simulink model "TflexDriver"  (R2018a)
settings: Solver=FixedStepAuto  StartTime=0.0  StopTime=inf  FixedStep=ts  RelTol=1e-3  EnableMultiTasking=on
values from neighbouring files (symbols this model uses):
  ts = 1/1000    (= 0.001)    [Tflex_PID_init.m]    (also in init.m = 0.00025; multisineInit.m)
libraries: xpcethercatlib x91, simulink x60
(part 1 of 2)
settings Model: SimulationMode=external  Creator=wout7  LastModifiedBy=wout7
settings SolverCC: ConcurrentTasks=on  AutoInsertRateTranBlk=on
settings DataIOCC: SaveFormat=StructureWithTime
settings OptimizationCC: BlockReduction=off  OptimizeBlockIOStorage=off  BufferReuse=off  GlobalBufferReuse=off  ExpressionFolding=off  LocalBlockOutputs=off  OptimizeDataStoreBuffers=off  BusAssignmentInplaceUpdate=off
settings HardwareCC: ProdBitPerPointer=32  ProdBitPerSizeT=32  ProdBitPerPtrDiffT=32  ProdLargestAtomicFloat=None  ProdWordSize=32  ProdLongLongMode=on  ProdHWDeviceType=Generic->32-bit x86 compatible
settings RTWCC: SystemTargetFile=slrt.tlc  TemplateMakefile=slrt_default_tmf  Description=Simulink Real-Time  CodeExecutionProfiling=on  RTWCompilerOptimization=on
settings SimulinkRealTimeCC: SupportVariableSizeSignals=on  RL32LogTETModifier=off  xPCConcurrentTasks=on

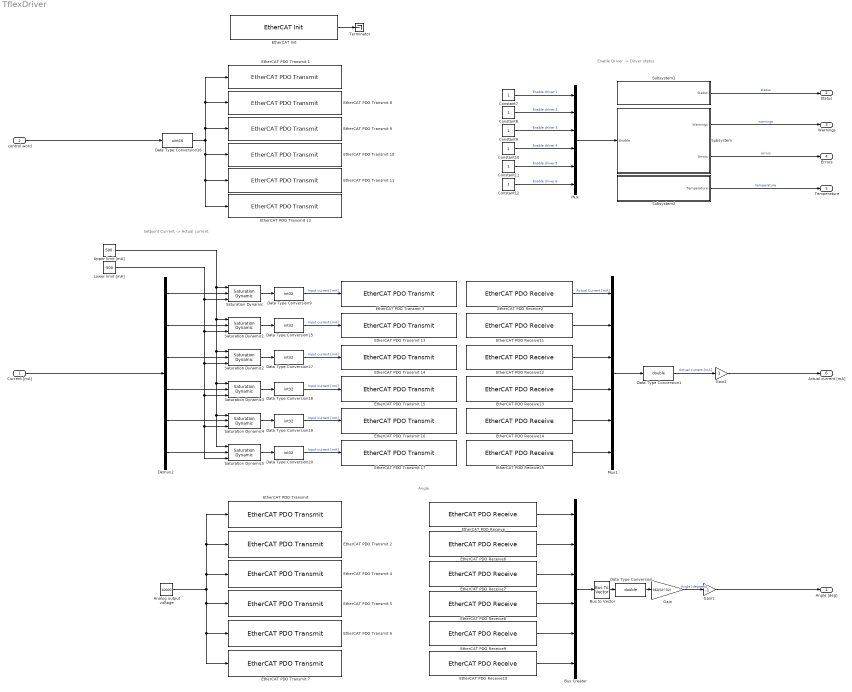
== system TflexDriver ==
  note: Angle
  note: Setpoint Current -> Actual current
  note: Enable Driver -> Dirver status
  Current [mA] : Inport
  control word : Inport  Port=2
  Analog output voltage : Constant  Value=10000  OutDataTypeStr=int16  SampleTime=-1
  Bus Creator : BusCreator  Inputs=6
  Bus to Vector : BusToVector
  Constant{7..12} (6 alike) : Constant  OutDataTypeStr=int32  SampleTime=1
  Data Type Conversion : DataTypeConversion  OutDataTypeStr=double
  Data Type Conversion1 : DataTypeConversion  OutDataTypeStr=double
  Data Type Conversion{9,15,17..20} (6 alike) : DataTypeConversion  OutDataTypeStr=int32
  Data Type Conversion16 : DataTypeConversion  OutDataTypeStr=uint16
  Demux2 : Demux  Outputs=6
  "EtherCAT Init " : xpcethercatlib/EtherCAT Init   Priority=0  config_file=C:\Users\wout7\Documents\GitHub\Inverse_dynamics_learning\TargetPC\6 DOF\pdo_mapping_6dr_1kHz.xml  device_id=0  pci_bus=13  pci_slot=0  pci_function=0  dctuning=0  enaDebug=off  enaDC=on  errLink=off  masterDbg=off  stateChgDbg=off  baseClock=off  masterCfg=off  logFile='c:\dbglog.txt'  sample_time=0.001000  DCMode=2
      settings: SourceProductName=Simulink Real-Time  SourceProductBaseCode=XP
  EtherCAT PDO Receive : xpcethercatlib/EtherCAT PDO Receive  Priority=2  sig_name=Drive 2 (AKD).Inputs_1.Position actual internal value  sig_offset=560  sig_type=int32  type_size=32  sig_dim=1  device_id=0  sample_time=0.001000
      settings: SourceProductName=Simulink Real-Time  SourceProductBaseCode=XP
  EtherCAT PDO Receive10 : xpcethercatlib/EtherCAT PDO Receive  Priority=2  sig_name=Drive 7 (AKD).Inputs_1.Position actual internal value  sig_offset=37488  sig_type=int32  type_size=32  sig_dim=1  device_id=0  sample_time=0.001000
      settings: SourceProductName=Simulink Real-Time  SourceProductBaseCode=XP
  EtherCAT PDO Receive11 : xpcethercatlib/EtherCAT PDO Receive  Priority=2  sig_name=Drive 3 (AKD).Inputs_1.Current actual value  sig_offset=12560  sig_type=int32  type_size=32  sig_dim=1  device_id=0  sample_time=0.001000
      settings: SourceProductName=Simulink Real-Time  SourceProductBaseCode=XP
  EtherCAT PDO Receive12 : xpcethercatlib/EtherCAT PDO Receive  Priority=2  sig_name=Drive 4 (AKD).Inputs_1.Current actual value  sig_offset=24848  sig_type=int32  type_size=32  sig_dim=1  device_id=0  sample_time=0.001000
      settings: SourceProductName=Simulink Real-Time  SourceProductBaseCode=XP
  EtherCAT PDO Receive13 : xpcethercatlib/EtherCAT PDO Receive  Priority=2  sig_name=Drive 5 (AKD).Inputs_1.Current actual value  sig_offset=37136  sig_type=int32  type_size=32  sig_dim=1  device_id=0  sample_time=0.001000
      settings: SourceProductName=Simulink Real-Time  SourceProductBaseCode=XP
  EtherCAT PDO Receive14 : xpcethercatlib/EtherCAT PDO Receive  Priority=2  sig_name=Drive 6 (AKD).Inputs_1.Current actual value  sig_offset=37296  sig_type=int32  type_size=32  sig_dim=1  device_id=0  sample_time=0.001000
      settings: SourceProductName=Simulink Real-Time  SourceProductBaseCode=XP
  EtherCAT PDO Receive15 : xpcethercatlib/EtherCAT PDO Receive  Priority=2  sig_name=Drive 7 (AKD).Inputs_1.Current actual value  sig_offset=37456  sig_type=int32  type_size=32  sig_dim=1  device_id=0  sample_time=0.001000
      settings: SourceProductName=Simulink Real-Time  SourceProductBaseCode=XP
  EtherCAT PDO Receive2 : xpcethercatlib/EtherCAT PDO Receive  Priority=2  sig_name=Drive 2 (AKD).Inputs_1.Current actual value  sig_offset=528  sig_type=int32  type_size=32  sig_dim=1  device_id=0  sample_time=0.001000
      settings: SourceProductName=Simulink Real-Time  SourceProductBaseCode=XP
  EtherCAT PDO Receive6 : xpcethercatlib/EtherCAT PDO Receive  Priority=2  sig_name=Drive 3 (AKD).Inputs_1.Position actual internal value  sig_offset=12592  sig_type=int32  type_size=32  sig_dim=1  device_id=0  sample_time=0.001000
      settings: SourceProductName=Simulink Real-Time  SourceProductBaseCode=XP
  EtherCAT PDO Receive7 : xpcethercatlib/EtherCAT PDO Receive  Priority=2  sig_name=Drive 4 (AKD).Inputs_1.Position actual internal value  sig_offset=24880  sig_type=int32  type_size=32  sig_dim=1  device_id=0  sample_time=0.001000
      settings: SourceProductName=Simulink Real-Time  SourceProductBaseCode=XP
  EtherCAT PDO Receive8 : xpcethercatlib/EtherCAT PDO Receive  Priority=2  sig_name=Drive 5 (AKD).Inputs_1.Position actual internal value  sig_offset=37168  sig_type=int32  type_size=32  sig_dim=1  device_id=0  sample_time=0.001000
      settings: SourceProductName=Simulink Real-Time  SourceProductBaseCode=XP
  EtherCAT PDO Receive9 : xpcethercatlib/EtherCAT PDO Receive  Priority=2  sig_name=Drive 6 (AKD).Inputs_1.Position actual internal value  sig_offset=37328  sig_type=int32  type_size=32  sig_dim=1  device_id=0  sample_time=0.001000
      settings: SourceProductName=Simulink Real-Time  SourceProductBaseCode=XP
  "EtherCAT PDO Transmit " : xpcethercatlib/EtherCAT PDO Transmit   Priority=3  sig_name=Drive 2 (AKD).Outputs.AOUT.VALUE write  sig_offset=480  sig_type=int16  type_size=16  sig_dim=1  device_id=0  sample_time=0.001000
      settings: SourceProductName=Simulink Real-Time  SourceProductBaseCode=XP
  EtherCAT PDO Transmit 1 : xpcethercatlib/EtherCAT PDO Transmit   Priority=3  sig_name=Drive 2 (AKD).Outputs.Controlword  sig_offset=464  sig_type=uint16  type_size=16  sig_dim=1  device_id=0  sample_time=0.001000
      settings: SourceProductName=Simulink Real-Time  SourceProductBaseCode=XP
  EtherCAT PDO Transmit 10 : xpcethercatlib/EtherCAT PDO Transmit   Priority=3  sig_name=Drive 5 (AKD).Outputs.Controlword  sig_offset=37072  sig_type=uint16  type_size=16  sig_dim=1  device_id=0  sample_time=0.001000
      settings: SourceProductName=Simulink Real-Time  SourceProductBaseCode=XP
  EtherCAT PDO Transmit 11 : xpcethercatlib/EtherCAT PDO Transmit   Priority=3  sig_name=Drive 6 (AKD).Outputs.Controlword  sig_offset=37232  sig_type=uint16  type_size=16  sig_dim=1  device_id=0  sample_time=0.001000
      settings: SourceProductName=Simulink Real-Time  SourceProductBaseCode=XP
  EtherCAT PDO Transmit 12 : xpcethercatlib/EtherCAT PDO Transmit   Priority=3  sig_name=Drive 7 (AKD).Outputs.Controlword  sig_offset=37392  sig_type=uint16  type_size=16  sig_dim=1  device_id=0  sample_time=0.001000
      settings: SourceProductName=Simulink Real-Time  SourceProductBaseCode=XP
  EtherCAT PDO Transmit 13 : xpcethercatlib/EtherCAT PDO Transmit   Priority=3  sig_name=Drive 3 (AKD).Outputs.Target current  sig_offset=12528  sig_type=int32  type_size=32  sig_dim=1  device_id=0  sample_time=0.001000
      settings: SourceProductName=Simulink Real-Time  SourceProductBaseCode=XP
  EtherCAT PDO Transmit 14 : xpcethercatlib/EtherCAT PDO Transmit   Priority=3  sig_name=Drive 4 (AKD).Outputs.Target current  sig_offset=24816  sig_type=int32  type_size=32  sig_dim=1  device_id=0  sample_time=0.001000
      settings: SourceProductName=Simulink Real-Time  SourceProductBaseCode=XP
  EtherCAT PDO Transmit 15 : xpcethercatlib/EtherCAT PDO Transmit   Priority=3  sig_name=Drive 5 (AKD).Outputs.Target current  sig_offset=37104  sig_type=int32  type_size=32  sig_dim=1  device_id=0  sample_time=0.001000
      settings: SourceProductName=Simulink Real-Time  SourceProductBaseCode=XP
  EtherCAT PDO Transmit 16 : xpcethercatlib/EtherCAT PDO Transmit   Priority=3  sig_name=Drive 6 (AKD).Outputs.Target current  sig_offset=37264  sig_type=int32  type_size=32  sig_dim=1  device_id=0  sample_time=0.001000
      settings: SourceProductName=Simulink Real-Time  SourceProductBaseCode=XP
  EtherCAT PDO Transmit 17 : xpcethercatlib/EtherCAT PDO Transmit   Priority=3  sig_name=Drive 7 (AKD).Outputs.Target current  sig_offset=37424  sig_type=int32  type_size=32  sig_dim=1  device_id=0  sample_time=0.001000
      settings: SourceProductName=Simulink Real-Time  SourceProductBaseCode=XP
  EtherCAT PDO Transmit 2 : xpcethercatlib/EtherCAT PDO Transmit   Priority=3  sig_name=Drive 3 (AKD).Outputs.AOUT.VALUE write  sig_offset=12512  sig_type=int16  type_size=16  sig_dim=1  device_id=0  sample_time=0.001000
      settings: SourceProductName=Simulink Real-Time  SourceProductBaseCode=XP
  EtherCAT PDO Transmit 3 : xpcethercatlib/EtherCAT PDO Transmit   Priority=3  sig_name=Drive 2 (AKD).Outputs.Target current  sig_offset=496  sig_type=int32  type_size=32  sig_dim=1  device_id=0  sample_time=0.001000
      settings: SourceProductName=Simulink Real-Time  SourceProductBaseCode=XP
  EtherCAT PDO Transmit 4 : xpcethercatlib/EtherCAT PDO Transmit   Priority=3  sig_name=Drive 4 (AKD).Outputs.AOUT.VALUE write  sig_offset=24800  sig_type=int16  type_size=16  sig_dim=1  device_id=0  sample_time=0.001000
      settings: SourceProductName=Simulink Real-Time  SourceProductBaseCode=XP
  EtherCAT PDO Transmit 5 : xpcethercatlib/EtherCAT PDO Transmit   Priority=3  sig_name=Drive 5 (AKD).Outputs.AOUT.VALUE write  sig_offset=37088  sig_type=int16  type_size=16  sig_dim=1  device_id=0  sample_time=0.001000
      settings: SourceProductName=Simulink Real-Time  SourceProductBaseCode=XP
  EtherCAT PDO Transmit 6 : xpcethercatlib/EtherCAT PDO Transmit   Priority=3  sig_name=Drive 6 (AKD).Outputs.AOUT.VALUE write  sig_offset=37248  sig_type=int16  type_size=16  sig_dim=1  device_id=0  sample_time=0.001000
      settings: SourceProductName=Simulink Real-Time  SourceProductBaseCode=XP
  EtherCAT PDO Transmit 7 : xpcethercatlib/EtherCAT PDO Transmit   Priority=3  sig_name=Drive 7 (AKD).Outputs.AOUT.VALUE write  sig_offset=37408  sig_type=int16  type_size=16  sig_dim=1  device_id=0  sample_time=0.001000
      settings: SourceProductName=Simulink Real-Time  SourceProductBaseCode=XP
  EtherCAT PDO Transmit 8 : xpcethercatlib/EtherCAT PDO Transmit   Priority=3  sig_name=Drive 3 (AKD).Outputs.Controlword  sig_offset=12496  sig_type=uint16  type_size=16  sig_dim=1  device_id=0  sample_time=0.001000
      settings: SourceProductName=Simulink Real-Time  SourceProductBaseCode=XP
  EtherCAT PDO Transmit 9 : xpcethercatlib/EtherCAT PDO Transmit   Priority=3  sig_name=Drive 4 (AKD).Outputs.Controlword  sig_offset=24784  sig_type=uint16  type_size=16  sig_dim=1  device_id=0  sample_time=0.001000
      settings: SourceProductName=Simulink Real-Time  SourceProductBaseCode=XP
  Gain : Gain  Gain=360/(2^32)
  Gain1 : Gain  Gain=-1
  Gain2 : Gain
  Lower limit [mA] : Constant  Value=-500  SampleTime=ts
  Mux : Mux  Inputs=6
  Mux1 : Mux  Inputs=6
  Saturation Dynamic{,1..5} (6 alike) : simulink/Discontinuities/Saturation Dynamic  OutMin=[]  OutMax=[]  OutDataTypeStr=Inherit: Same as second input  OutDataType=fixdt(1, 16)  OutScaling=2^-10  DoSatur=off
  Subsystem : Subsystem
  Subsystem1 : Subsystem
  Subsystem2 : Subsystem
  Terminator : Terminator
  Upper limit [mA] : Constant  Value=500  SampleTime=ts
  Angle [deg] : Outport
  Status : Outport  Port=2
  Warnings : Outport  Port=3
  Errors : Outport  Port=4
  Temperature : Outport  Port=5
  Actual current [mA] : Outport  Port=6
  wires:
  Lower limit [mA]/1 -> Saturation Dynamic/3, Saturation Dynamic1/3, Saturation Dynamic2/3, Saturation Dynamic3/3, Saturation Dynamic4/3, Saturation Dynamic5/3
  Data Type Conversion17/1 -> EtherCAT PDO Transmit 14/1  "Input current [mA]"
  Data Type Conversion/1 -> Gain/1
  Constant7/1 -> Mux/1  "Enable driver 1"
  EtherCAT PDO Receive10/1 -> Bus Creator/6
  Analog output voltage/1 -> EtherCAT PDO Transmit 7/1, EtherCAT PDO Transmit 6/1, EtherCAT PDO Transmit 5/1, "EtherCAT PDO Transmit "/1, EtherCAT PDO Transmit 2/1, EtherCAT PDO Transmit 4/1
  Subsystem1/1(Status) -> Status/1  "status"
  Constant12/1 -> Mux/6  "Enable driver 6"
  EtherCAT PDO Receive2/1 -> Mux1/1  "Actual Current [mA]"
  Mux/1 -> Subsystem/1(Enable)
  Subsystem/1(Warnings) -> Warnings/1  "warnings"
  Saturation Dynamic1/1 -> Data Type Conversion15/1
  EtherCAT PDO Receive11/1 -> Mux1/2
  Gain1/1 -> Angle [deg]/1
  Gain2/1 -> Actual current [mA]/1
  control word/1 -> Data Type Conversion16/1
  Current [mA]/1 -> Demux2/1
  Data Type Conversion16/1 -> EtherCAT PDO Transmit 1/1, EtherCAT PDO Transmit 8/1, EtherCAT PDO Transmit 9/1, EtherCAT PDO Transmit 12/1, EtherCAT PDO Transmit 11/1, EtherCAT PDO Transmit 10/1
  Gain/1 -> Gain1/1  "Angle [degrees]"
  Subsystem2/1(Temperature) -> Temperature/1  "temperature"
  Demux2/6 -> Saturation Dynamic5/2
  Demux2/3 -> Saturation Dynamic2/2
  Saturation Dynamic5/1 -> Data Type Conversion20/1
  Demux2/2 -> Saturation Dynamic1/2
  Upper limit [mA]/1 -> Saturation Dynamic3/1, Saturation Dynamic4/1, Saturation Dynamic5/1, Saturation Dynamic2/1, Saturation Dynamic1/1, Saturation Dynamic/1
  Saturation Dynamic2/1 -> Data Type Conversion17/1
  Bus to Vector/1 -> Data Type Conversion/1
  Mux1/1 -> Data Type Conversion1/1
  Constant9/1 -> Mux/3  "Enable driver 3"
  Data Type Conversion15/1 -> EtherCAT PDO Transmit 13/1  "Input current [mA]"
  Data Type Conversion19/1 -> EtherCAT PDO Transmit 16/1  "Input current [mA]"
  EtherCAT PDO Receive7/1 -> Bus Creator/3
  Data Type Conversion20/1 -> EtherCAT PDO Transmit 17/1  "Input current [mA]"
  EtherCAT PDO Receive/1 -> Bus Creator/1
  Demux2/5 -> Saturation Dynamic4/2
  Bus Creator/1 -> Bus to Vector/1
  Data Type Conversion1/1 -> Gain2/1  "Actual current [mA]"
  EtherCAT PDO Receive14/1 -> Mux1/5
  Constant10/1 -> Mux/4  "Enable driver 4"
  Constant11/1 -> Mux/5  "Enable driver 5"
  Demux2/1 -> Saturation Dynamic/2
  EtherCAT PDO Receive9/1 -> Bus Creator/5
  Data Type Conversion9/1 -> EtherCAT PDO Transmit 3/1  "Input current [mA]"
  Constant8/1 -> Mux/2  "Enable driver 2"
  EtherCAT PDO Receive13/1 -> Mux1/4
  EtherCAT PDO Receive12/1 -> Mux1/3
  Saturation Dynamic4/1 -> Data Type Conversion19/1
  Demux2/4 -> Saturation Dynamic3/2
  Data Type Conversion18/1 -> EtherCAT PDO Transmit 15/1  "Input current [mA]"
  EtherCAT PDO Receive6/1 -> Bus Creator/2
  EtherCAT PDO Receive8/1 -> Bus Creator/4
  EtherCAT PDO Receive15/1 -> Mux1/6
  Subsystem/2(Errors) -> Errors/1  "errors"
  Saturation Dynamic/1 -> Data Type Conversion9/1
  "EtherCAT Init "/1 -> Terminator/1
  Saturation Dynamic3/1 -> Data Type Conversion18/1

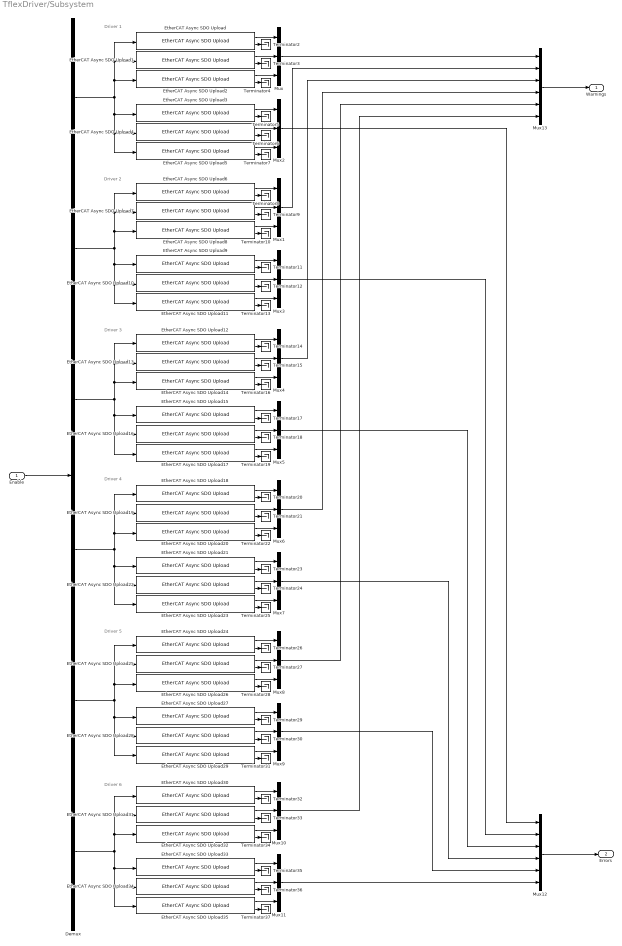
== system TflexDriver/Subsystem ==
  note: Driver 1
  note: Driver 2
  note: Driver 3
  note: Driver 4
  note: Driver 5
  note: Driver 6
  Enable : Inport
  Demux : Demux  Outputs=6
  EtherCAT Async SDO Upload : xpcethercatlib/EtherCAT Async SDO Upload  index=8192  subIndex=1  sig_type=uint32  sig_dim=1  device_id=0  slave_name=Drive 2 (AKD)  sample_time=1  slave_addr=1001  selected_slave=Term 1 (EK1100)  timeout=500  slave_found=1
      settings: SourceProductName=Simulink Real-Time  SourceProductBaseCode=XP
  EtherCAT Async SDO Upload1 : xpcethercatlib/EtherCAT Async SDO Upload  index=8192  subIndex=2  sig_type=uint32  sig_dim=1  device_id=0  slave_name=Drive 2 (AKD)  sample_time=1  slave_addr=1001  selected_slave=Term 1 (EK1100)  timeout=500  slave_found=1
      settings: SourceProductName=Simulink Real-Time  SourceProductBaseCode=XP
  EtherCAT Async SDO Upload10 : xpcethercatlib/EtherCAT Async SDO Upload  index=8193  subIndex=2  sig_type=uint32  sig_dim=1  device_id=0  slave_name=Drive 3 (AKD)  sample_time=1  slave_addr=1002  selected_slave=Term 1 (EK1100)  timeout=500  slave_found=1
      settings: SourceProductName=Simulink Real-Time  SourceProductBaseCode=XP
  EtherCAT Async SDO Upload11 : xpcethercatlib/EtherCAT Async SDO Upload  index=8193  subIndex=3  sig_type=uint32  sig_dim=1  device_id=0  slave_name=Drive 3 (AKD)  sample_time=1  slave_addr=1002  selected_slave=Term 1 (EK1100)  timeout=500  slave_found=1
      settings: SourceProductName=Simulink Real-Time  SourceProductBaseCode=XP
  EtherCAT Async SDO Upload12 : xpcethercatlib/EtherCAT Async SDO Upload  index=8192  subIndex=1  sig_type=uint32  sig_dim=1  device_id=0  slave_name=Drive 4 (AKD)  sample_time=1  slave_addr=1003  selected_slave=Term 1 (EK1100)  timeout=500  slave_found=1
      settings: SourceProductName=Simulink Real-Time  SourceProductBaseCode=XP
  EtherCAT Async SDO Upload13 : xpcethercatlib/EtherCAT Async SDO Upload  index=8192  subIndex=2  sig_type=uint32  sig_dim=1  device_id=0  slave_name=Drive 4 (AKD)  sample_time=1  slave_addr=1003  selected_slave=Term 1 (EK1100)  timeout=500  slave_found=1
      settings: SourceProductName=Simulink Real-Time  SourceProductBaseCode=XP
  EtherCAT Async SDO Upload14 : xpcethercatlib/EtherCAT Async SDO Upload  index=8192  subIndex=3  sig_type=uint32  sig_dim=1  device_id=0  slave_name=Drive 4 (AKD)  sample_time=1  slave_addr=1003  selected_slave=Term 1 (EK1100)  timeout=500  slave_found=1
      settings: SourceProductName=Simulink Real-Time  SourceProductBaseCode=XP
  EtherCAT Async SDO Upload15 : xpcethercatlib/EtherCAT Async SDO Upload  index=8193  subIndex=1  sig_type=uint32  sig_dim=1  device_id=0  slave_name=Drive 4 (AKD)  sample_time=1  slave_addr=1003  selected_slave=Term 1 (EK1100)  timeout=500  slave_found=1
      settings: SourceProductName=Simulink Real-Time  SourceProductBaseCode=XP
  EtherCAT Async SDO Upload16 : xpcethercatlib/EtherCAT Async SDO Upload  index=8193  subIndex=2  sig_type=uint32  sig_dim=1  device_id=0  slave_name=Drive 4 (AKD)  sample_time=1  slave_addr=1003  selected_slave=Term 1 (EK1100)  timeout=500  slave_found=1
      settings: SourceProductName=Simulink Real-Time  SourceProductBaseCode=XP
  EtherCAT Async SDO Upload17 : xpcethercatlib/EtherCAT Async SDO Upload  index=8193  subIndex=3  sig_type=uint32  sig_dim=1  device_id=0  slave_name=Drive 4 (AKD)  sample_time=1  slave_addr=1003  selected_slave=Term 1 (EK1100)  timeout=500  slave_found=1
      settings: SourceProductName=Simulink Real-Time  SourceProductBaseCode=XP
  EtherCAT Async SDO Upload18 : xpcethercatlib/EtherCAT Async SDO Upload  index=8192  subIndex=1  sig_type=uint32  sig_dim=1  device_id=0  slave_name=Drive 5 (AKD)  sample_time=1  slave_addr=1004  selected_slave=Term 1 (EK1100)  timeout=500  slave_found=1
      settings: SourceProductName=Simulink Real-Time  SourceProductBaseCode=XP
  EtherCAT Async SDO Upload19 : xpcethercatlib/EtherCAT Async SDO Upload  index=8192  subIndex=2  sig_type=uint32  sig_dim=1  device_id=0  slave_name=Drive 5 (AKD)  sample_time=1  slave_addr=1004  selected_slave=Term 1 (EK1100)  timeout=500  slave_found=1
      settings: SourceProductName=Simulink Real-Time  SourceProductBaseCode=XP
  EtherCAT Async SDO Upload2 : xpcethercatlib/EtherCAT Async SDO Upload  index=8192  subIndex=3  sig_type=uint32  sig_dim=1  device_id=0  slave_name=Drive 1 (AKD)  sample_time=1  slave_addr=1001  selected_slave=Term 1 (EK1100)  timeout=500  slave_found=1
      settings: SourceProductName=Simulink Real-Time  SourceProductBaseCode=XP
  EtherCAT Async SDO Upload20 : xpcethercatlib/EtherCAT Async SDO Upload  index=8192  subIndex=3  sig_type=uint32  sig_dim=1  device_id=0  slave_name=Drive 5 (AKD)  sample_time=1  slave_addr=1004  selected_slave=Term 1 (EK1100)  timeout=500  slave_found=1
      settings: SourceProductName=Simulink Real-Time  SourceProductBaseCode=XP
  EtherCAT Async SDO Upload21 : xpcethercatlib/EtherCAT Async SDO Upload  index=8193  subIndex=1  sig_type=uint32  sig_dim=1  device_id=0  slave_name=Drive 5 (AKD)  sample_time=1  slave_addr=1004  selected_slave=Term 1 (EK1100)  timeout=500  slave_found=1
      settings: SourceProductName=Simulink Real-Time  SourceProductBaseCode=XP
  EtherCAT Async SDO Upload22 : xpcethercatlib/EtherCAT Async SDO Upload  index=8193  subIndex=2  sig_type=uint32  sig_dim=1  device_id=0  slave_name=Drive 5 (AKD)  sample_time=1  slave_addr=1004  selected_slave=Term 1 (EK1100)  timeout=500  slave_found=1
      settings: SourceProductName=Simulink Real-Time  SourceProductBaseCode=XP
  EtherCAT Async SDO Upload23 : xpcethercatlib/EtherCAT Async SDO Upload  index=8193  subIndex=3  sig_type=uint32  sig_dim=1  device_id=0  slave_name=Drive 5 (AKD)  sample_time=1  slave_addr=1004  selected_slave=Term 1 (EK1100)  timeout=500  slave_found=1
      settings: SourceProductName=Simulink Real-Time  SourceProductBaseCode=XP
  EtherCAT Async SDO Upload24 : xpcethercatlib/EtherCAT Async SDO Upload  index=8192  subIndex=1  sig_type=uint32  sig_dim=1  device_id=0  slave_name=Drive 6 (AKD)  sample_time=1  slave_addr=1005  selected_slave=Term 1 (EK1100)  timeout=500  slave_found=1
      settings: SourceProductName=Simulink Real-Time  SourceProductBaseCode=XP
  EtherCAT Async SDO Upload25 : xpcethercatlib/EtherCAT Async SDO Upload  index=8192  subIndex=2  sig_type=uint32  sig_dim=1  device_id=0  slave_name=Drive 6 (AKD)  sample_time=1  slave_addr=1005  selected_slave=Term 1 (EK1100)  timeout=500  slave_found=1
      settings: SourceProductName=Simulink Real-Time  SourceProductBaseCode=XP
  EtherCAT Async SDO Upload26 : xpcethercatlib/EtherCAT Async SDO Upload  index=8192  subIndex=3  sig_type=uint32  sig_dim=1  device_id=0  slave_name=Drive 6 (AKD)  sample_time=1  slave_addr=1005  selected_slave=Term 1 (EK1100)  timeout=500  slave_found=1
      settings: SourceProductName=Simulink Real-Time  SourceProductBaseCode=XP
  EtherCAT Async SDO Upload27 : xpcethercatlib/EtherCAT Async SDO Upload  index=8193  subIndex=1  sig_type=uint32  sig_dim=1  device_id=0  slave_name=Drive 6 (AKD)  sample_time=1  slave_addr=1005  selected_slave=Term 1 (EK1100)  timeout=500  slave_found=1
      settings: SourceProductName=Simulink Real-Time  SourceProductBaseCode=XP
  EtherCAT Async SDO Upload28 : xpcethercatlib/EtherCAT Async SDO Upload  index=8193  subIndex=2  sig_type=uint32  sig_dim=1  device_id=0  slave_name=Drive 6 (AKD)  sample_time=1  slave_addr=1005  selected_slave=Term 1 (EK1100)  timeout=500  slave_found=1
      settings: SourceProductName=Simulink Real-Time  SourceProductBaseCode=XP
  EtherCAT Async SDO Upload29 : xpcethercatlib/EtherCAT Async SDO Upload  index=8193  subIndex=3  sig_type=uint32  sig_dim=1  device_id=0  slave_name=Drive 6 (AKD)  sample_time=1  slave_addr=1005  selected_slave=Term 1 (EK1100)  timeout=500  slave_found=1
      settings: SourceProductName=Simulink Real-Time  SourceProductBaseCode=XP
  EtherCAT Async SDO Upload3 : xpcethercatlib/EtherCAT Async SDO Upload  index=8193  subIndex=1  sig_type=uint32  sig_dim=1  device_id=0  slave_name=""  sample_time=1  slave_addr=0  selected_slave=Term 1 (EK1100)  timeout=500  slave_found=1
      settings: SourceProductName=Simulink Real-Time  SourceProductBaseCode=XP
  EtherCAT Async SDO Upload30 : xpcethercatlib/EtherCAT Async SDO Upload  index=8192  subIndex=1  sig_type=uint32  sig_dim=1  device_id=0  slave_name=Drive 7 (AKD)  sample_time=1  slave_addr=1006  selected_slave=Term 1 (EK1100)  timeout=500  slave_found=1
      settings: SourceProductName=Simulink Real-Time  SourceProductBaseCode=XP
  EtherCAT Async SDO Upload31 : xpcethercatlib/EtherCAT Async SDO Upload  index=8192  subIndex=2  sig_type=uint32  sig_dim=1  device_id=0  slave_name=Drive 7 (AKD)  sample_time=1  slave_addr=1006  selected_slave=Term 1 (EK1100)  timeout=500  slave_found=1
      settings: SourceProductName=Simulink Real-Time  SourceProductBaseCode=XP
  EtherCAT Async SDO Upload32 : xpcethercatlib/EtherCAT Async SDO Upload  index=8192  subIndex=3  sig_type=uint32  sig_dim=1  device_id=0  slave_name=Drive 7 (AKD)  sample_time=1  slave_addr=1006  selected_slave=Term 1 (EK1100)  timeout=500  slave_found=1
      settings: SourceProductName=Simulink Real-Time  SourceProductBaseCode=XP
  EtherCAT Async SDO Upload33 : xpcethercatlib/EtherCAT Async SDO Upload  index=8193  subIndex=1  sig_type=uint32  sig_dim=1  device_id=0  slave_name=Drive 7 (AKD)  sample_time=1  slave_addr=1006  selected_slave=Term 1 (EK1100)  timeout=500  slave_found=1
      settings: SourceProductName=Simulink Real-Time  SourceProductBaseCode=XP
  EtherCAT Async SDO Upload34 : xpcethercatlib/EtherCAT Async SDO Upload  index=8193  subIndex=2  sig_type=uint32  sig_dim=1  device_id=0  slave_name=Drive 7 (AKD)  sample_time=1  slave_addr=1006  selected_slave=Term 1 (EK1100)  timeout=500  slave_found=1
      settings: SourceProductName=Simulink Real-Time  SourceProductBaseCode=XP
  EtherCAT Async SDO Upload35 : xpcethercatlib/EtherCAT Async SDO Upload  index=8193  subIndex=3  sig_type=uint32  sig_dim=1  device_id=0  slave_name=Drive 7 (AKD)  sample_time=1  slave_addr=1006  selected_slave=Term 1 (EK1100)  timeout=500  slave_found=1
      settings: SourceProductName=Simulink Real-Time  SourceProductBaseCode=XP
  EtherCAT Async SDO Upload4 : xpcethercatlib/EtherCAT Async SDO Upload  index=8193  subIndex=2  sig_type=uint32  sig_dim=1  device_id=0  slave_name=Drive 2 (AKD)  sample_time=1  slave_addr=1001  selected_slave=Term 1 (EK1100)  timeout=500  slave_found=1
      settings: SourceProductName=Simulink Real-Time  SourceProductBaseCode=XP
  EtherCAT Async SDO Upload5 : xpcethercatlib/EtherCAT Async SDO Upload  index=8193  subIndex=3  sig_type=uint32  sig_dim=1  device_id=0  slave_name=Drive 1 (AKD)  sample_time=1  slave_addr=1001  selected_slave=Term 1 (EK1100)  timeout=500  slave_found=1
      settings: SourceProductName=Simulink Real-Time  SourceProductBaseCode=XP
  EtherCAT Async SDO Upload6 : xpcethercatlib/EtherCAT Async SDO Upload  index=8192  subIndex=1  sig_type=uint32  sig_dim=1  device_id=0  slave_name=Drive 3 (AKD)  sample_time=1  slave_addr=1002  selected_slave=Term 1 (EK1100)  timeout=500  slave_found=1
      settings: SourceProductName=Simulink Real-Time  SourceProductBaseCode=XP
  EtherCAT Async SDO Upload7 : xpcethercatlib/EtherCAT Async SDO Upload  index=8192  subIndex=2  sig_type=uint32  sig_dim=1  device_id=0  slave_name=Drive 3 (AKD)  sample_time=1  slave_addr=1002  selected_slave=Term 1 (EK1100)  timeout=500  slave_found=1
      settings: SourceProductName=Simulink Real-Time  SourceProductBaseCode=XP
  EtherCAT Async SDO Upload8 : xpcethercatlib/EtherCAT Async SDO Upload  index=8192  subIndex=3  sig_type=uint32  sig_dim=1  device_id=0  slave_name=Drive 3 (AKD)  sample_time=1  slave_addr=1002  selected_slave=Term 1 (EK1100)  timeout=500  slave_found=1
      settings: SourceProductName=Simulink Real-Time  SourceProductBaseCode=XP
  EtherCAT Async SDO Upload9 : xpcethercatlib/EtherCAT Async SDO Upload  index=8193  subIndex=1  sig_type=uint32  sig_dim=1  device_id=0  slave_name=Drive 3 (AKD)  sample_time=1  slave_addr=1002  selected_slave=Term 1 (EK1100)  timeout=500  slave_found=1
      settings: SourceProductName=Simulink Real-Time  SourceProductBaseCode=XP
  Mux{,1..11} (12 alike) : Mux  Inputs=3
  Mux12 : Mux  Inputs=6
  Mux13 : Mux  Inputs=6
  Terminator{2..37} (36 alike) : Terminator
  Warnings : Outport
  Errors : Outport  Port=2
  wires:
  EtherCAT Async SDO Upload13/2 -> Terminator15/1
  EtherCAT Async SDO Upload23/2 -> Terminator25/1
  EtherCAT Async SDO Upload25/2 -> Terminator27/1
  EtherCAT Async SDO Upload9/2 -> Terminator11/1
  EtherCAT Async SDO Upload5/2 -> Terminator7/1
  EtherCAT Async SDO Upload30/2 -> Terminator32/1
  EtherCAT Async SDO Upload27/2 -> Terminator29/1
  EtherCAT Async SDO Upload12/2 -> Terminator14/1
  EtherCAT Async SDO Upload24/2 -> Terminator26/1
  EtherCAT Async SDO Upload26/2 -> Terminator28/1
  Mux4/1 -> Mux13/3
  Demux/3 -> EtherCAT Async SDO Upload12/1, EtherCAT Async SDO Upload13/1, EtherCAT Async SDO Upload14/1, EtherCAT Async SDO Upload17/1, EtherCAT Async SDO Upload16/1, EtherCAT Async SDO Upload15/1
  EtherCAT Async SDO Upload30/1 -> Mux10/1
  Demux/2 -> EtherCAT Async SDO Upload11/1, EtherCAT Async SDO Upload10/1, EtherCAT Async SDO Upload9/1, EtherCAT Async SDO Upload6/1, EtherCAT Async SDO Upload7/1, EtherCAT Async SDO Upload8/1
  EtherCAT Async SDO Upload9/1 -> Mux3/1
  EtherCAT Async SDO Upload18/2 -> Terminator20/1
  EtherCAT Async SDO Upload8/2 -> Terminator10/1
  EtherCAT Async SDO Upload11/2 -> Terminator13/1
  Demux/6 -> EtherCAT Async SDO Upload30/1, EtherCAT Async SDO Upload31/1, EtherCAT Async SDO Upload32/1, EtherCAT Async SDO Upload35/1, EtherCAT Async SDO Upload34/1, EtherCAT Async SDO Upload33/1
  Demux/4 -> EtherCAT Async SDO Upload18/1, EtherCAT Async SDO Upload19/1, EtherCAT Async SDO Upload20/1, EtherCAT Async SDO Upload23/1, EtherCAT Async SDO Upload22/1, EtherCAT Async SDO Upload21/1
  EtherCAT Async SDO Upload19/2 -> Terminator21/1
  Mux11/1 -> Mux12/6
  Demux/1 -> EtherCAT Async SDO Upload5/1, EtherCAT Async SDO Upload4/1, EtherCAT Async SDO Upload3/1, EtherCAT Async SDO Upload/1, EtherCAT Async SDO Upload1/1, EtherCAT Async SDO Upload2/1
  EtherCAT Async SDO Upload15/2 -> Terminator17/1
  Mux6/1 -> Mux13/4
  EtherCAT Async SDO Upload34/2 -> Terminator36/1
  Demux/5 -> EtherCAT Async SDO Upload24/1, EtherCAT Async SDO Upload25/1, EtherCAT Async SDO Upload26/1, EtherCAT Async SDO Upload29/1, EtherCAT Async SDO Upload28/1, EtherCAT Async SDO Upload27/1
  EtherCAT Async SDO Upload6/2 -> Terminator8/1
  EtherCAT Async SDO Upload/1 -> Mux/1
  EtherCAT Async SDO Upload7/2 -> Terminator9/1
  EtherCAT Async SDO Upload16/2 -> Terminator18/1
  Mux5/1 -> Mux12/3
  EtherCAT Async SDO Upload10/2 -> Terminator12/1
  EtherCAT Async SDO Upload35/2 -> Terminator37/1
  EtherCAT Async SDO Upload21/1 -> Mux7/1
  Mux8/1 -> Mux13/5
  EtherCAT Async SDO Upload31/2 -> Terminator33/1
  EtherCAT Async SDO Upload32/1 -> Mux10/3
  EtherCAT Async SDO Upload15/1 -> Mux5/1
  EtherCAT Async SDO Upload/2 -> Terminator2/1
  EtherCAT Async SDO Upload13/1 -> Mux4/2
  EtherCAT Async SDO Upload33/2 -> Terminator35/1
  EtherCAT Async SDO Upload4/2 -> Terminator6/1
  EtherCAT Async SDO Upload28/2 -> Terminator30/1
  EtherCAT Async SDO Upload1/2 -> Terminator3/1
  Mux1/1 -> Mux13/2
  EtherCAT Async SDO Upload8/1 -> Mux1/3
  EtherCAT Async SDO Upload19/1 -> Mux6/2
  EtherCAT Async SDO Upload20/2 -> Terminator22/1
  EtherCAT Async SDO Upload12/1 -> Mux4/1
  EtherCAT Async SDO Upload29/2 -> Terminator31/1
  EtherCAT Async SDO Upload2/1 -> Mux/3
  EtherCAT Async SDO Upload26/1 -> Mux8/3
  EtherCAT Async SDO Upload22/2 -> Terminator24/1
  EtherCAT Async SDO Upload28/1 -> Mux9/2
  Mux/1 -> Mux13/1
  EtherCAT Async SDO Upload3/2 -> Terminator5/1
  Mux9/1 -> Mux12/5
  EtherCAT Async SDO Upload2/2 -> Terminator4/1
  EtherCAT Async SDO Upload33/1 -> Mux11/1
  EtherCAT Async SDO Upload17/1 -> Mux5/3
  EtherCAT Async SDO Upload31/1 -> Mux10/2
  EtherCAT Async SDO Upload27/1 -> Mux9/1
  EtherCAT Async SDO Upload1/1 -> Mux/2
  EtherCAT Async SDO Upload3/1 -> Mux2/1
  EtherCAT Async SDO Upload11/1 -> Mux3/3
  EtherCAT Async SDO Upload7/1 -> Mux1/2
  EtherCAT Async SDO Upload6/1 -> Mux1/1
  EtherCAT Async SDO Upload34/1 -> Mux11/2
  Mux10/1 -> Mux13/6
  EtherCAT Async SDO Upload22/1 -> Mux7/2
  EtherCAT Async SDO Upload23/1 -> Mux7/3
  EtherCAT Async SDO Upload18/1 -> Mux6/1
  EtherCAT Async SDO Upload10/1 -> Mux3/2
  EtherCAT Async SDO Upload14/1 -> Mux4/3
  EtherCAT Async SDO Upload35/1 -> Mux11/3
  EtherCAT Async SDO Upload24/1 -> Mux8/1
  EtherCAT Async SDO Upload20/1 -> Mux6/3
  Mux2/1 -> Mux12/1
  EtherCAT Async SDO Upload4/1 -> Mux2/2
  EtherCAT Async SDO Upload25/1 -> Mux8/2
  EtherCAT Async SDO Upload16/1 -> Mux5/2
  Mux7/1 -> Mux12/4
  Mux3/1 -> Mux12/2
  EtherCAT Async SDO Upload5/1 -> Mux2/3
  EtherCAT Async SDO Upload32/2 -> Terminator34/1
  EtherCAT Async SDO Upload29/1 -> Mux9/3
  EtherCAT Async SDO Upload14/2 -> Terminator16/1
  EtherCAT Async SDO Upload17/2 -> Terminator19/1
  EtherCAT Async SDO Upload21/2 -> Terminator23/1
  Mux12/1 -> Errors/1
  Mux13/1 -> Warnings/1
  Enable/1 -> Demux/1
